simulink model "ros_image_filters_0704"  (R2017a)
settings: Solver=FixedStepDiscrete  StartTime=0.0  StopTime=inf  FixedStep=0.01  RelTol=1e-3  EnableMultiTasking=on
model workspace (MAT data in the model file):
  SL_ROS_VariableLengthArrays_MaxSizes.CommonInfo.ArrayTruncateAction = 'EmitWarning'
  SL_ROS_VariableLengthArrays_MaxSizes.MsgTypeMap = containers.Map
  SL_ROS_VariableLengthArrays_MaxSizes.MsgTypeMap.serialization.keys = {'sensor_msgs/Image'}
  SL_ROS_VariableLengthArrays_MaxSizes.MsgTypeMap.serialization.values{1}(1).PropertyName = 'Data'
  SL_ROS_VariableLengthArrays_MaxSizes.MsgTypeMap.serialization.values{1}(1).DataType = 'uint8'
  SL_ROS_VariableLengthArrays_MaxSizes.MsgTypeMap.serialization.values{1}(1).MaxLength = 1555200
  SL_ROS_VariableLengthArrays_MaxSizes.MsgTypeMap.serialization.values{1}(2).PropertyName = 'Encoding'
  SL_ROS_VariableLengthArrays_MaxSizes.MsgTypeMap.serialization.values{1}(2).DataType = 'uint8'
  SL_ROS_VariableLengthArrays_MaxSizes.MsgTypeMap.serialization.values{1}(2).MaxLength = 4
  SL_ROS_VariableLengthArrays_MaxSizes.MsgTypeMap.serialization.uniformity = 0
  SL_ROS_VariableLengthArrays_MaxSizes.MsgTypeMap.serialization.keyType = 'char'
  SL_ROS_VariableLengthArrays_MaxSizes.MsgTypeMap.serialization.valueType = 'any'
  blockSize = [270 480]
undefined symbols (not defined in the file): Rec, SDTV, strel
libraries: robotlib x7, visionconversions x5, visionsinks x5, simulink x3, visionmorphops x2, visionfilter x1, visionanalysis x1
settings Model: Creator=qifan  LastModifiedBy=qifan
settings SolverCC: AutoInsertRateTranBlk=on
settings DataIOCC: SaveOutput=off  SaveTime=off
settings OptimizationCC: PassReuseOutputArgsAs=Individual arguments  StateBitsets=on  DataBitsets=on  ZeroExternalMemoryAtStartup=off  ZeroInternalMemoryAtStartup=off  NoFixptDivByZeroProtection=on  LifeSpan=1  MaxStackSize=64
settings DebuggingCC: ParameterTunabilityLossMsg=error
settings HardwareCC: ProdBitPerPointer=32  ProdBitPerSizeT=32  ProdBitPerPtrDiffT=32  ProdLargestAtomicFloat=None  ProdIntDivRoundTo=Undefined  ProdEndianess=Unspecified  ProdWordSize=32  ProdHWDeviceType=Generic->Unspecified (assume 32-bit Generic)
settings SFSimCC: MATLABDynamicMemAlloc=off
settings RTWCC: SystemTargetFile=ert.tlc  HardwareBoard=Robot Operating System (ROS)  TLCOptions="-p0 -aInlineSetEventsForThisBaseRateFcn=TLC_FALSE -aSuppressMultiTaskScheduler=TLC_FALSE  -aRateBasedStepFcn=0"  GenCodeOnly=on  TemplateMakefile=ert_default_tmf  Description=Embedded Coder  GenerateReport=on  RTWVerbose=off  Toolchain=Catkin  IncludeHyperlinkInReport=on  LaunchReport=on  TargetLang=C++  GenerateTraceInfo=on  GenerateTraceReport=on  GenerateTraceReportSl=on  GenerateTraceReportSf=on  GenerateTraceReportEml=on
settings CodeAppCC: ForceParamTrailComments=on  IgnoreCustomStorageClasses=off  OperatorAnnotations=on  SimulinkDataObjDesc=on  SFDataObjDesc=on  MATLABFcnDesc=on  CustomSymbolStrGlobalVar=rt$N$M  CustomSymbolStrType=$N$M  CustomSymbolStrFcn=$N$M$F  CustomSymbolStrMacro=$N$M  InsertBlockDesc=on  MATLABSourceComments=on
settings ERTTargetCC: CodeReplacementLibrary=ISO_C  SupportNonFinite=off  SupportComplex=off  SupportContinuousTime=on  RootIOFormat=Structure reference

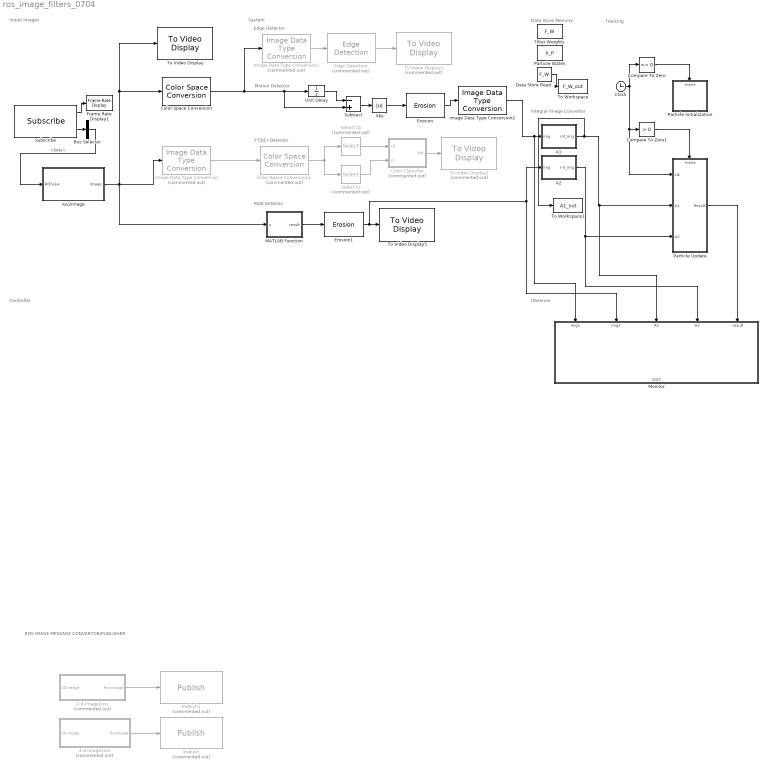
== system ros_image_filters_0704 ==
  note: Integral Image
      | Converter
  note: Observer
  note: Controller
  note: Imput Images
  note: System
  note: Y'CbCr Detector
  note: RGB Detector
  note: Edge Detector
  note: Motion Detector
  note: Data Store Memory
  note: Tracking
  note: ROS IMAGE MESSAGE CONVERTOR/PUBLISHER
  2-d-image2ros : Subsystem  Commented=on
  3-d-image2ros : Subsystem  Commented=on
  A1 : MATLAB Function  TreatAsAtomicUnit=on
  A2 : MATLAB Function  TreatAsAtomicUnit=on
  Abs : Abs
  Bus Selector : BusSelector  OutputSignals=Data
  Clock : Clock
  Color Classifier : Subsystem  Commented=on
  Color Space Conversion : visionconversions/Color Space  Conversion  conversion=Obsolete  conversionActive=R'G'B' to intensity  wp_str=D65  rec=Rec. 601 (SDTV)  sys=1125/60/2:1  imagePorts=One multidimensional signal
      settings: SourceProductName=Computer Vision System Toolbox
  Color Space Conversion1 : visionconversions/Color Space  Conversion  Commented=on  conversion=Obsolete  conversionActive=R'G'B' to Y'CbCr  wp_str=D65  rec=Rec. 601 (SDTV)  sys=1125/60/2:1  imagePorts=One multidimensional signal
      settings: SourceProductName=Computer Vision System Toolbox
  Compare To Zero : simulink/Logic and Bit Operations/Compare To Zero  relop=<=  OutDataTypeStr=boolean
  Compare To Zero1 : simulink/Logic and Bit Operations/Compare To Zero  relop=>  OutDataTypeStr=uint8
  Data Store Read : DataStoreRead  DataStoreName=F_W
  Edge Detection : visionanalysis/Edge Detection  Commented=on  method=Sobel  outputType=Binary image  userDefinedThreshold=off  thresholdSource=Input port  threshold=20  thresholdTuning=4  edgeThinning=off  threshold_canny=[0.25 0.60]  autoPercent=70  sigma=1  prodOutputMode=Binary point scaling  prodOutputWordLength=32  prodOutputFracLength=8  roundingMode=Floor  overflowMode=off
      settings: SourceProductName=Computer Vision System Toolbox  SourceProductBaseCode=VP
  Erosion : visionmorphops/Erosion  nhoodsrc=Specify via dialog  strel=strel('square',7)
      settings: SourceProductName=Computer Vision System Toolbox  SourceProductBaseCode=VP
  Erosion1 : visionmorphops/Erosion  nhoodsrc=Specify via dialog  strel=strel('square',7)
      settings: SourceProductName=Computer Vision System Toolbox  SourceProductBaseCode=VP
  Filter Weights : DataStoreMemory  DataStoreName=F_W  ReadBeforeWriteMsg=warning  WriteAfterWriteMsg=warning  WriteAfterReadMsg=warning  InitialValue=[0.5,0.5,0,0,0,0,0,0]  ShowAdditionalParam=off  OutDataTypeStr=double
  Frame Rate Display1 : visionsinks/Frame Rate Display  UpdateRate=10
      settings: SourceProductName=Computer Vision System Toolbox  SourceProductBaseCode=VP
  Image Data Type Conversion : visionconversions/Image Data Type Conversion  Commented=on  outDT=single  isSigned=on  wordLen=16  numFracBits=0
      settings: SourceProductName=Computer Vision System Toolbox  SourceProductBaseCode=VP
  Image Data Type Conversion1 : visionconversions/Image Data Type Conversion  Commented=on  outDT=single  isSigned=on  wordLen=16  numFracBits=0
      settings: SourceProductName=Computer Vision System Toolbox  SourceProductBaseCode=VP
  Image Data Type Conversion2 : visionconversions/Image Data Type Conversion  outDT=double  isSigned=on  wordLen=16  numFracBits=0
      settings: SourceProductName=Computer Vision System Toolbox  SourceProductBaseCode=VP
  MATLAB Function : MATLAB Function  TreatAsAtomicUnit=on
  Monitor : Subsystem
  Particle Initialization : Subsystem
  Particle States : DataStoreMemory  DataStoreName=X_P  ReadBeforeWriteMsg=warning  WriteAfterWriteMsg=warning  WriteAfterReadMsg=warning  InitialValue=zeros(200,3,2)  ShowAdditionalParam=off  OutDataTypeStr=double
  Particle Update : Subsystem
  Publish : robotlib/Publish  Commented=on  SourceLibraryInfo=This block requires Robotics System Toolbox  topicSource=Specify your own  topic=/image_color  messageType=sensor_msgs/Image  messageQueueLength=1
      settings: SourceProductBaseCode=RO
  Publish1 : robotlib/Publish  Commented=on  SourceLibraryInfo=This block requires Robotics System Toolbox  topicSource=Specify your own  topic=/image_erode  messageType=sensor_msgs/Image  messageQueueLength=1
      settings: SourceProductBaseCode=RO
  Select Cb : Selector  Commented=on  NumberOfDimensions=3  InputPortWidth=3  IndexOptions=Select all,Select all,Index vector (dialog)  Indices=[1 3],1,2  OutputSizes=1,1,1
  Select Cr : Selector  Commented=on  NumberOfDimensions=3  InputPortWidth=3  IndexOptions=Select all,Select all,Index vector (dialog)  Indices=[1 3],1,3  OutputSizes=1,1,1
  Subscribe : robotlib/Subscribe  SourceLibraryInfo=This block requires Robotics System Toolbox  topicSource=Specify your own  topic=/image_bridge  messageType=sensor_msgs/Image  sampleTime=-1  messageQueueLength=1
      settings: SourceProductBaseCode=RO
  Subtract : Sum  Inputs=-+
  To Video Display : visionsinks/To Video Display  windowSizeMode=Normal  openAtMdlStart=on  fullScreen=off  videoWindowX=160  videoWindowY=130  saveWindowSize=off  videoWindowWidth=960  videoWindowHeight=540  inputColorFormat=RGB  inputType=Obsolete  imagePorts=One multidimensional signal  OutputDevice=On-screen video monitor  dataOrg=Column-major  isWindowOpen=off
      settings: SourceProductName=Computer Vision System Toolbox
  To Video Display1 : visionsinks/To Video Display  Commented=on  windowSizeMode=Normal  openAtMdlStart=on  fullScreen=off  videoWindowX=260  videoWindowY=97  saveWindowSize=off  videoWindowWidth=962  videoWindowHeight=542  inputColorFormat=RGB  inputType=Obsolete  imagePorts=One multidimensional signal  OutputDevice=On-screen video monitor  dataOrg=Column-major  isWindowOpen=off
      settings: SourceProductName=Computer Vision System Toolbox
  To Video Display2 : visionsinks/To Video Display  Commented=on  windowSizeMode=Normal  openAtMdlStart=on  fullScreen=off  videoWindowX=184  videoWindowY=153  saveWindowSize=off  videoWindowWidth=960  videoWindowHeight=540  inputColorFormat=RGB  inputType=Obsolete  imagePorts=One multidimensional signal  OutputDevice=On-screen video monitor  dataOrg=Column-major  isWindowOpen=off
      settings: SourceProductName=Computer Vision System Toolbox
  To Video Display5 : visionsinks/To Video Display  windowSizeMode=Normal  openAtMdlStart=on  fullScreen=off  videoWindowX=260  videoWindowY=97  saveWindowSize=off  videoWindowWidth=962  videoWindowHeight=542  inputColorFormat=RGB  inputType=Obsolete  imagePorts=One multidimensional signal  OutputDevice=On-screen video monitor  dataOrg=Column-major  isWindowOpen=off
      settings: SourceProductName=Computer Vision System Toolbox
  To Workspace : ToWorkspace  VariableName=F_W_out  SaveFormat=Timeseries  SampleTime=-1
  To Workspace1 : ToWorkspace  VariableName=A1_out  SaveFormat=Timeseries  SampleTime=-1
  Unit Delay : UnitDelay  SampleTime=-1
  ros2image : Subsystem
  wires:
  Subscribe/1 -> Frame Rate Display1/1
  Bus Selector/1 -> ros2image/1(ROSraw)  "<Data>"
  Subscribe/2 -> Bus Selector/1
  Color Space Conversion/1 -> Unit Delay/1, Subtract/2, Image Data Type Conversion1/1
  3-d-image2ros/1(RosImage) -> Publish/1
  2-d-image2ros/1(Ros-image) -> Publish1/1
  Color Space Conversion1/1 -> Select Cr/1, Select Cb/1
  Select Cb/1 -> Color Classifier/1(cb)
  Select Cr/1 -> Color Classifier/2(cr)
  Color Classifier/1(BW) -> To Video Display1/1
  Image Data Type Conversion/1 -> Color Space Conversion1/1
  Edge Detection/1 -> To Video Display2/1
  Image Data Type Conversion1/1 -> Edge Detection/1
  Unit Delay/1 -> Subtract/1
  Subtract/1 -> Abs/1
  Abs/1 -> Erosion/1
  Erosion/1 -> Image Data Type Conversion2/1
  MATLAB Function/1(result) -> Erosion1/1
  Clock/1 -> Compare To Zero1/1, Particle Update/1(clk), Compare To Zero/1
  Compare To Zero/1 -> Particle Initialization/Enable
  Compare To Zero1/1 -> Particle Update/Enable
  Erosion1/1 -> A2/1(img), Monitor/2(img2), To Video Display5/1
  ros2image/1(Image) -> MATLAB Function/1(u), Image Data Type Conversion/1, Color Space Conversion/1, To Video Display/1
  Particle Update/1(Result) -> Monitor/5(result)
  A1/1(int_img) -> To Workspace1/1, Particle Update/2(A1), Monitor/3("A1 ")
  A2/1(int_img) -> Particle Update/3(A2), Monitor/4(A2)
  Image Data Type Conversion2/1 -> Monitor/1(img1), A1/1(img)
  Data Store Read/1 -> To Workspace/1

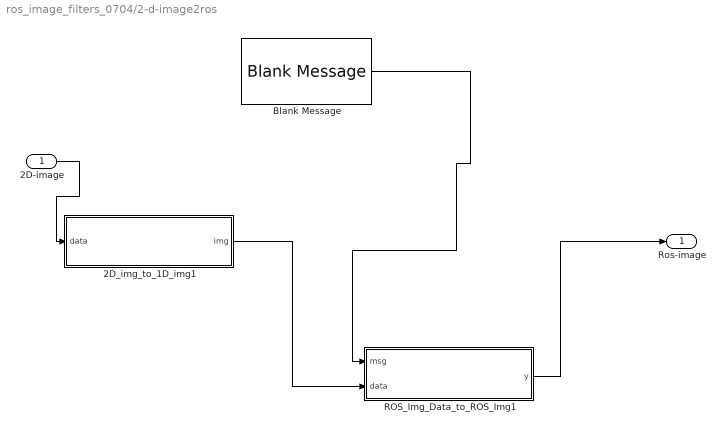
== system ros_image_filters_0704/2-d-image2ros ==
  2D-image : Inport
  2D_img_to_1D_img1 : MATLAB Function  TreatAsAtomicUnit=on
  Blank Message : robotlib/Blank Message  SourceLibraryInfo=This block requires Robotics System Toolbox  messageType=sensor_msgs/Image  SampleTime=inf
      settings: SourceProductBaseCode=RO
  ROS_Img_Data_to_ROS_Img1 : MATLAB Function  TreatAsAtomicUnit=on
  Ros-image : Outport
  wires:
  2D-image/1 -> 2D_img_to_1D_img1/1(data)
  ROS_Img_Data_to_ROS_Img1/1(y) -> Ros-image/1
  Blank Message/1 -> ROS_Img_Data_to_ROS_Img1/1(msg)
  2D_img_to_1D_img1/1(img) -> ROS_Img_Data_to_ROS_Img1/2(data)

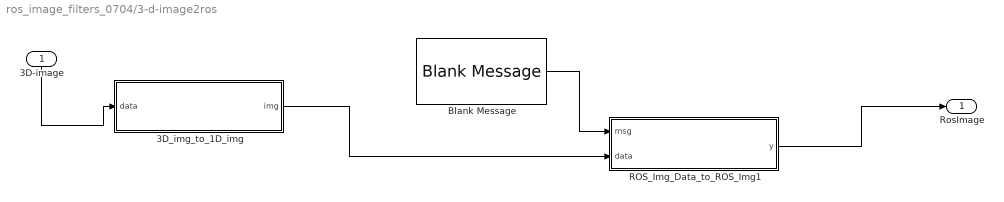
== system ros_image_filters_0704/3-d-image2ros ==
  3D-image : Inport
  3D_img_to_1D_img : MATLAB Function  TreatAsAtomicUnit=on
  Blank Message : robotlib/Blank Message  SourceLibraryInfo=This block requires Robotics System Toolbox  messageType=sensor_msgs/Image  SampleTime=inf
      settings: SourceProductBaseCode=RO
  ROS_Img_Data_to_ROS_Img1 : MATLAB Function  TreatAsAtomicUnit=on
  RosImage : Outport
  wires:
  3D-image/1 -> 3D_img_to_1D_img/1(data)
  ROS_Img_Data_to_ROS_Img1/1(y) -> RosImage/1
  Blank Message/1 -> ROS_Img_Data_to_ROS_Img1/1(msg)
  3D_img_to_1D_img/1(img) -> ROS_Img_Data_to_ROS_Img1/2(data)

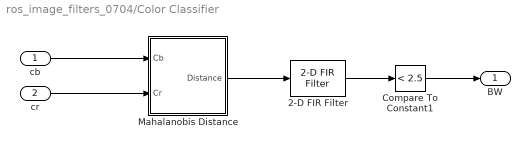
== system ros_image_filters_0704/Color Classifier ==
  cb : Inport
  cr : Inport  Port=2
  2-D FIR Filter : visionfilter/2-D FIR Filter  separable=off  filtSrc=Specify via dialog  filterMtrx=single(1/9*ones(3))  verticalFilter=[4 0]  horizontalFilter=[4 0]  outSize=Full  padType=Constant  padSrc=Specify via dialog  padVal=0  method=Convolution  firstCoeffSignedness=Signed  firstCoeffDataTypeStr=Inherit: Same word length as input  firstCoeffLastDataTypeStr=Inherit: Same word length as input  firstCoeffMin=[]  firstCoeffMax=[]  outputMode=Binary point scaling  outputWordLength=32  outputFracLength=12  outputSignedness=Auto  outputDataTypeStr=fixdt([],32,12)  outputLastDataTypeStr=fixdt([],32,12)  outputMin=[]  outputMax=[]  accumDataTypeStr=Inherit: Same as product output  accumLastDataTypeStr=Inherit: Same as product output  prodOutputMode=Binary point scaling  prodOutputWordLength=32  prodOutputFracLength=10  prodOutputDataTypeStr=fixdt([],32,10)  prodOutputLastDataTypeStr=fixdt([],32,10)  roundingMode=Floor  overflowMode=off
      settings: SourceProductName=Computer Vision System Toolbox  SourceProductBaseCode=VP
  Compare To Constant1 : simulink/Logic and Bit Operations/Compare To Constant  relop=<  const=2.5  OutDataTypeStr=boolean  ZeroCross=off
  "Mahalanobis Distance " : Subsystem
  BW : Outport
  wires:
  "Mahalanobis Distance "/1(Distance) -> 2-D FIR Filter/1
  cb/1 -> "Mahalanobis Distance "/1(Cb)
  cr/1 -> "Mahalanobis Distance "/2(Cr)
  Compare To Constant1/1 -> BW/1
  2-D FIR Filter/1 -> Compare To Constant1/1

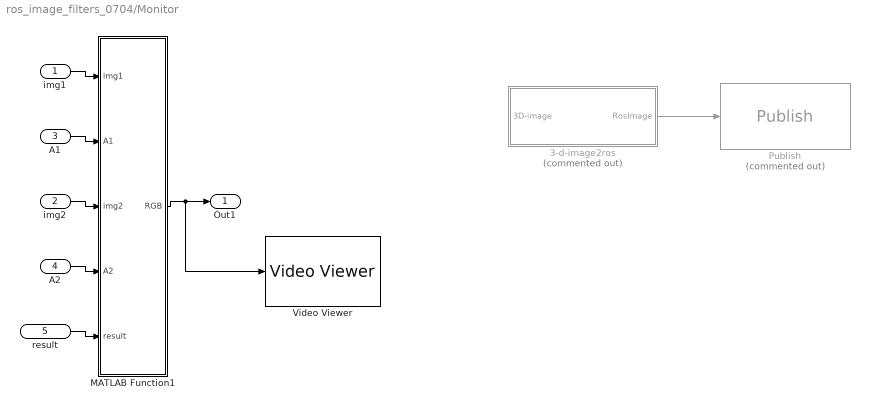
== system ros_image_filters_0704/Monitor ==
  img1 : Inport
  img2 : Inport  Port=2
  "A1 " : Inport  Port=3
  A2 : Inport  Port=4
  result : Inport  Port=5
  3-d-image2ros : Subsystem  Commented=on
  MATLAB Function1 : MATLAB Function  TreatAsAtomicUnit=on
  Publish : robotlib/Publish  Commented=on  SourceLibraryInfo=This block requires Robotics System Toolbox  topicSource=Specify your own  topic=/tracking_result  messageType=sensor_msgs/Image  messageQueueLength=1
      settings: SourceProductBaseCode=RO
  Video Viewer : VideoViewer  FigPos=[58 798 1223 693]
  Out1 : Outport
  wires:
  MATLAB Function1/1(RGB) -> Video Viewer/1, Out1/1
  result/1 -> MATLAB Function1/5(result)
  "A1 "/1 -> MATLAB Function1/2(A1)
  A2/1 -> MATLAB Function1/4(A2)
  img1/1 -> MATLAB Function1/1(img1)
  img2/1 -> MATLAB Function1/3(img2)
  3-d-image2ros/1(RosImage) -> Publish/1

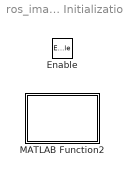
== system ros_image_filters_0704/Particle Initialization ==
  Enable : EnablePort
  MATLAB Function2 : MATLAB Function  TreatAsAtomicUnit=on

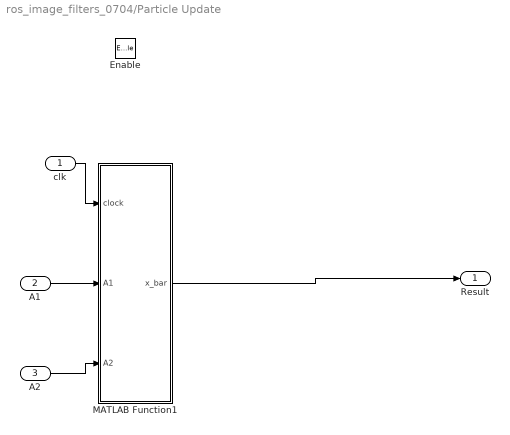
== system ros_image_filters_0704/Particle Update ==
  clk : Inport
  A1 : Inport  Port=2
  A2 : Inport  Port=3
  Enable : EnablePort
  MATLAB Function1 : MATLAB Function  TreatAsAtomicUnit=on
  Result : Outport
  wires:
  clk/1 -> MATLAB Function1/1(clock)
  MATLAB Function1/1(x_bar) -> Result/1
  A1/1 -> MATLAB Function1/2(A1)
  A2/1 -> MATLAB Function1/3(A2)

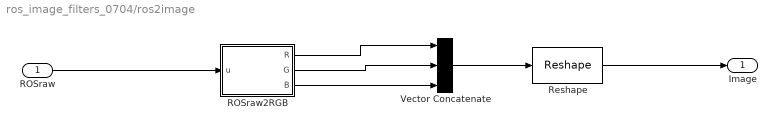
== system ros_image_filters_0704/ros2image ==
  ROSraw : Inport  PortDimensions=1555200
  ROSraw2RGB : MATLAB Function  TreatAsAtomicUnit=on
  Reshape : Reshape  OutputDimensionality=Customize  OutputDimensions=[540,960,3]
  Vector Concatenate : Concatenate  NumInputs=3  Mode=Multidimensional array  ConcatenateDimension=2
  Image : Outport
  wires:
  ROSraw2RGB/3(B) -> Vector Concatenate/3
  ROSraw2RGB/1(R) -> Vector Concatenate/1
  Reshape/1 -> Image/1
  ROSraw/1 -> ROSraw2RGB/1(u)
  ROSraw2RGB/2(G) -> Vector Concatenate/2
  Vector Concatenate/1 -> Reshape/1

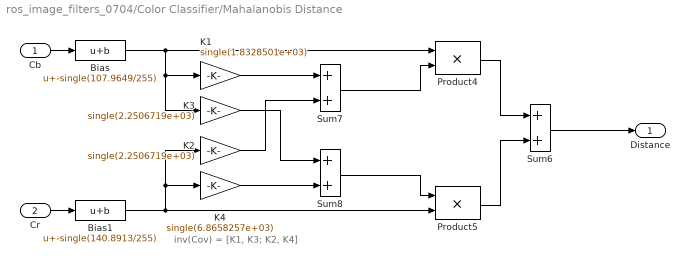
== system ros_image_filters_0704/Color Classifier/Mahalanobis Distance  ==
  note: inv(Cov) = [K1, K3; K2, K4]
  Cb : Inport
  Cr : Inport  Port=2
  Bias : Bias  Bias=-single(107.9649/255)
  Bias1 : Bias  Bias=-single(140.8913/255)
  K1 : Gain  Gain=single(1.8328501e+03)  SaturateOnIntegerOverflow=on  OutDataTypeStr=Inherit: Same as input  ParamDataTypeStr=Inherit: Same as input
  K2 : Gain  Gain=single(2.2506719e+03)  SaturateOnIntegerOverflow=on  OutDataTypeStr=Inherit: Same as input  ParamDataTypeStr=Inherit: Same as input
  K3 : Gain  Gain=single(2.2506719e+03)  SaturateOnIntegerOverflow=on  OutDataTypeStr=Inherit: Same as input  ParamDataTypeStr=Inherit: Same as input
  K4 : Gain  Gain=single(6.8658257e+03)  SaturateOnIntegerOverflow=on  OutDataTypeStr=Inherit: Same as input  ParamDataTypeStr=Inherit: Same as input
  Product4 : Product  SaturateOnIntegerOverflow=on  InputSameDT=on  OutDataTypeStr=Inherit: Same as first input
  Product5 : Product  SaturateOnIntegerOverflow=on  InputSameDT=on  OutDataTypeStr=Inherit: Same as first input
  Sum6 : Sum  SaturateOnIntegerOverflow=on  InputSameDT=on  OutDataTypeStr=Inherit: Same as first input
  Sum7 : Sum  SaturateOnIntegerOverflow=on  InputSameDT=on  OutDataTypeStr=Inherit: Same as first input
  Sum8 : Sum  SaturateOnIntegerOverflow=on  InputSameDT=on  OutDataTypeStr=Inherit: Same as first input
  Distance : Outport
  wires:
  Cb/1 -> Bias/1
  Cr/1 -> Bias1/1
  K4/1 -> Sum8/2
  Product4/1 -> Sum6/1
  Product5/1 -> Sum6/2
  K1/1 -> Sum7/1
  K2/1 -> Sum7/2
  K3/1 -> Sum8/1
  Sum7/1 -> Product4/2
  Sum8/1 -> Product5/1
  Bias/1 -> Product4/1, K1/1, K3/1
  Bias1/1 -> Product5/2, K4/1, K2/1
  Sum6/1 -> Distance/1

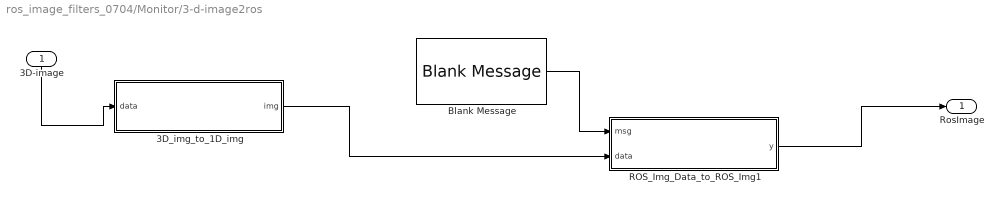
== system ros_image_filters_0704/Monitor/3-d-image2ros ==
  3D-image : Inport
  3D_img_to_1D_img : MATLAB Function  TreatAsAtomicUnit=on
  Blank Message : robotlib/Blank Message  SourceLibraryInfo=This block requires Robotics System Toolbox  messageType=sensor_msgs/Image  SampleTime=inf
      settings: SourceProductBaseCode=RO
  ROS_Img_Data_to_ROS_Img1 : MATLAB Function  TreatAsAtomicUnit=on
  RosImage : Outport
  wires:
  3D-image/1 -> 3D_img_to_1D_img/1(data)
  ROS_Img_Data_to_ROS_Img1/1(y) -> RosImage/1
  Blank Message/1 -> ROS_Img_Data_to_ROS_Img1/1(msg)
  3D_img_to_1D_img/1(img) -> ROS_Img_Data_to_ROS_Img1/2(data)

== matlab function ros_image_filters_0704/3-d-image2ros/ROS_Img_Data_to_ROS_Img1 ==
  data: msg input; y output Bus: SL_Bus_ros_image_filters_0619_sensor_msgs_Image; data input size=1555200
function y = rosImgData2rosImg(msg, data)
% assignString - Assign a string in a ROS message
%
% MSG = assignString(blankMsg) assigns a known string value to a 
%  string field in a ROS message, and outputs the updated ROS message.
%
%  blankMsg (input): A bus for a 'std_msgs/String' message. This is 
%      used to initialize the output. 
%  msg (output): A bus for a 'std_msgs/String' message, with the Data 
%      field set to a string.

%   Copyright 2015 The MathWorks, Inc.
%#codegen

% Note: The datatype of 'msg' has been explicitly set to the appropriate 
% Simulink bus type ("Bus: SL_Bus_robotROSMessageUsageExample_std_msgs_String"). 
%
% If the model name is changed, the datatype needs to be changed as well:
%   1) Click "Edit Data" in the Editor toolstrip to open "Ports and Data Manager"
%   2) Select "msg". From the "Type" dropdown, select "--- Refresh data types ---"
%   3) Set datatype to "Bus: SL_Bus_<modelname>_std_msgs_String"
    
stringToAssign = 'rgb8';
height = 540;
width = 960;

% msg (std_msgs/String) consists of
%           Data : array of type uint8
%   Data_SL_Info : struct with fields CurrentLength, ReceivedLength
msg.Encoding = uint8(stringToAssign)';
msg.Encoding_SL_Info.CurrentLength = uint32(length(stringToAssign));

msg.Data = uint8(data);
msg.Data_SL_Info.CurrentLength = uint32(length(data));

msg.Height = uint32(height);
msg.Width = uint32(width);
msg.Step = uint32(width * 3);

y = msg;

== matlab function ros_image_filters_0704/3-d-image2ros/3D_img_to_1D_img ==
  data: img output uint8; data input
function img = threeD_img_to_1D_img(data)
% assignString - Assign a string in a ROS message
%
% MSG = assignString(blankMsg) assigns a known string value to a 
%  string field in a ROS message, and outputs the updated ROS message.
%
%  blankMsg (input): A bus for a 'std_msgs/String' message. This is 
%      used to initialize the output. 
%  msg (output): A bus for a 'std_msgs/String' message, with the Data 
%      field set to a string.

%   Copyright 2015 The MathWorks, Inc.
%#codegen

% Note: The datatype of 'msg' has been explicitly set to the appropriate 
% Simulink bus type ("Bus: SL_Bus_robotROSMessageUsageExample_std_msgs_String"). 
%
% If the model name is changed, the datatype needs to be changed as well:
%   1) Click "Edit Data" in the Editor toolstrip to open "Ports and Data Manager"
%   2) Select "msg". From the "Type" dropdown, select "--- Refresh data types ---"
%   3) Set datatype to "Bus: SL_Bus_<modelname>_std_msgs_String"
    

% msg (std_msgs/String) consists of
%           Data : array of type uint8
%   Data_SL_Info : struct with fields CurrentLength, ReceivedLength
img = uint8(zeros(1, 1555200));
img(1:3:end) = data(:,:,1)';
img(2:3:end) = data(:,:,2)';
img(3:3:end) = data(:,:,3)';

== matlab function ros_image_filters_0704/MATLAB Function ==
  data: u input; result output
function result = fcn(u)

R = u(:, :, 1);
G = u(:, :, 2);
B = u(:, :, 3);


result = double(zeros(540, 960, 1));

%result(:, :, 1) = R./(R + G + B);
%result(:, :, 2) = G./(R + G + B);
%result(:, :, 3) = B./(R + G + B);


for i = 1:540
    for j = 1:960
        rgb = u(i, j, :);
        if rgb(1) > 95 && rgb(2) > 40 && rgb(3) > 20 && max(rgb) - min(rgb) > 15 ...
            && abs(rgb(1) - rgb(2)) > 15 && rgb(1) > rgb(2) && rgb(1) > rgb(3)
            result(i, j) = 1;
        end
    end
end

== matlab function ros_image_filters_0704/2-d-image2ros/2D_img_to_1D_img1 ==
  data: img output uint8; data input
function img = twoD_img_to_1D_img(data)
% assignString - Assign a string in a ROS message
%
% MSG = assignString(blankMsg) assigns a known string value to a 
%  string field in a ROS message, and outputs the updated ROS message.
%
%  blankMsg (input): A bus for a 'std_msgs/String' message. This is 
%      used to initialize the output. 
%  msg (output): A bus for a 'std_msgs/String' message, with the Data 
%      field set to a string.

%   Copyright 2015 The MathWorks, Inc.
%#codegen

% Note: The datatype of 'msg' has been explicitly set to the appropriate 
% Simulink bus type ("Bus: SL_Bus_robotROSMessageUsageExample_std_msgs_String"). 
%
% If the model name is changed, the datatype needs to be changed as well:
%   1) Click "Edit Data" in the Editor toolstrip to open "Ports and Data Manager"
%   2) Select "msg". From the "Type" dropdown, select "--- Refresh data types ---"
%   3) Set datatype to "Bus: SL_Bus_<modelname>_std_msgs_String"
    

% msg (std_msgs/String) consists of
%           Data : array of type uint8
%   Data_SL_Info : struct with fields CurrentLength, ReceivedLength
img = uint8(zeros(1, 1555200));
img(1:3:end) = data';
img(2:3:end) = data';
img(3:3:end) = data';

== matlab function ros_image_filters_0704/2-d-image2ros/ROS_Img_Data_to_ROS_Img1 ==
  data: msg input; y output Bus: SL_Bus_ros_image_filters_0619_sensor_msgs_Image; data input size=1555200
function y = rosImgData2rosImg(msg, data)
% assignString - Assign a string in a ROS message
%
% MSG = assignString(blankMsg) assigns a known string value to a 
%  string field in a ROS message, and outputs the updated ROS message.
%
%  blankMsg (input): A bus for a 'std_msgs/String' message. This is 
%      used to initialize the output. 
%  msg (output): A bus for a 'std_msgs/String' message, with the Data 
%      field set to a string.

%   Copyright 2015 The MathWorks, Inc.
%#codegen

% Note: The datatype of 'msg' has been explicitly set to the appropriate 
% Simulink bus type ("Bus: SL_Bus_robotROSMessageUsageExample_std_msgs_String"). 
%
% If the model name is changed, the datatype needs to be changed as well:
%   1) Click "Edit Data" in the Editor toolstrip to open "Ports and Data Manager"
%   2) Select "msg". From the "Type" dropdown, select "--- Refresh data types ---"
%   3) Set datatype to "Bus: SL_Bus_<modelname>_std_msgs_String"
    
stringToAssign = 'rgb8';
height = 540;
width = 960;

% msg (std_msgs/String) consists of
%           Data : array of type uint8
%   Data_SL_Info : struct with fields CurrentLength, ReceivedLength
msg.Encoding = uint8(stringToAssign)';
msg.Encoding_SL_Info.CurrentLength = uint32(length(stringToAssign));

msg.Data = uint8(data);
msg.Data_SL_Info.CurrentLength = uint32(length(data));

msg.Height = uint32(height);
msg.Width = uint32(width);
msg.Step = uint32(width * 3);

y = msg;

== matlab function ros_image_filters_0704/ros2image/ROSraw2RGB ==
  data: u input; R output; G output; B output
function [R,G,B] = fcn(u)
%#codegen
Rs = u(1:3:end);
Gs = u(2:3:end);
Bs = u(3:3:end);
B = reshape(Rs,960,540)';
G = reshape(Gs,960,540)';
R = reshape(Bs,960,540)';

== matlab function ros_image_filters_0704/Particle Update/MATLAB Function1 ==
  data: clock input; X_P data_store_memory; x_bar output; A1 input; A2 input
function x_bar = fcn(clock,A1,A2)

coder.extrinsic('imshow');
global X_P;


N = 200; % sample population

W_pre = X_P(:, 3, 2); % weights of old sample
S_new = zeros(N, 3, 2); % initial new sample container

s_k_pre = randsample(N,N,true,W_pre); % Sampling from previous state

%disp(s_k_pre);

for i = 1:N
    index = s_k_pre(i);
    p_top_left = reshape(X_P(index, 1, :), [1 2]); % get sample position
    
    s_v = reshape(X_P(index, 2, :),[1 2]);% get sample velocity
    s_width = X_P(index, 3, 1);% get sample width
    
    p_inrange_1 = [1, 1] < p_top_left;
    p_inrange_2 = p_top_left <= [540 - s_width, 960 - s_width];
    if sum([p_inrange_1 p_inrange_2]) ~= 4
        p_top_left = [rand * (540 - s_width), rand * (960 - s_width)];
    end

    p_tl = ceil(p_top_left);
    p_tr = ceil(p_top_left + [0, s_width]);
    p_bl = ceil(p_top_left + [s_width, 0]);
    p_br = ceil(p_top_left + [s_width, s_width]);
    
    value = A1(p_tl(1), p_tl(2)) + A1(p_br(1),p_br(2))...
    - A1(p_tr(1), p_tr(2)) - A1(p_bl(1),p_bl(2)); % update new weight

    w_new = value;
    
    if value < 1
        p_top_left = [rand * (540 - s_width), rand * (960 - s_width)];
        w_new = value + 0.01;
    end
    
    s_v_new = s_v + [randn, randn] * 5; % update velocity
    % s_width_new = s_width + randn; % update width
    p_new = p_top_left + s_v + randn;
    
    S_new(i, :, :) = [p_new; s_v_new; s_width, w_new];
end



[~, max_index] = max(X_P(:, 3, 2));
%RGB = insertMarker(image,int16(reshape([S_new(:,1,2), S_new(:,1,1)], [200, 2])),'o','color',[255 0 0],...
%    'size', 10);
%%% !!!!!!!!!!!!!!RGB = insertShape(img1, 'FilledCircle', [int16([S_new(max_index, 1, 2), S_new(max_index, 1, 1)]),10]);
x_bar = reshape(X_P(max_index, :, :), [3 2]);
X_P = S_new;
%disp(x_bar);
%disp(size(x_bar));


%RGB = insertMarker(RGB, reshape([S_new(:,1,2),S_new(:,1,1)], [N 2]),'o','color','green','size',10);


%imshow(image);
%hold on;
%[max_weight max_index] = max(S_new(:, 3, 2));
%plot(S_new(:,1,2),S_new(:,1,1),'r.','MarkerSize',20);
%plot(S_new(max_index, 1, 2), S_new(max_index, 1, 1), 'g.', 'MarkerSize', 100);
%hold off;

== matlab function ros_image_filters_0704/Particle Initialization/MATLAB Function2 ==
  data: X_P data_store_memory
function fcn

global X_P;


N = 200;


for i = 1:N
    weight = 1 / N;
    width = 50;
    
    X_P(i,2,:) = [0, 0];
    X_P(i,3,:) = [width, weight];
    x = rand * 540;
    y = rand * 960;
    X_P(i,1,:) = [x, y];
end

== matlab function ros_image_filters_0704/Monitor/3-d-image2ros/3D_img_to_1D_img ==
  data: img output uint8; data input
function img = threeD_img_to_1D_img(data)
% assignString - Assign a string in a ROS message
%
% MSG = assignString(blankMsg) assigns a known string value to a 
%  string field in a ROS message, and outputs the updated ROS message.
%
%  blankMsg (input): A bus for a 'std_msgs/String' message. This is 
%      used to initialize the output. 
%  msg (output): A bus for a 'std_msgs/String' message, with the Data 
%      field set to a string.

%   Copyright 2015 The MathWorks, Inc.
%#codegen

% Note: The datatype of 'msg' has been explicitly set to the appropriate 
% Simulink bus type ("Bus: SL_Bus_robotROSMessageUsageExample_std_msgs_String"). 
%
% If the model name is changed, the datatype needs to be changed as well:
%   1) Click "Edit Data" in the Editor toolstrip to open "Ports and Data Manager"
%   2) Select "msg". From the "Type" dropdown, select "--- Refresh data types ---"
%   3) Set datatype to "Bus: SL_Bus_<modelname>_std_msgs_String"
    

% msg (std_msgs/String) consists of
%           Data : array of type uint8
%   Data_SL_Info : struct with fields CurrentLength, ReceivedLength
img = uint8(zeros(1, 1555200));
img(1:3:end) = data(:,:,1)';
img(2:3:end) = data(:,:,2)';
img(3:3:end) = data(:,:,3)';

== matlab function ros_image_filters_0704/Monitor/3-d-image2ros/ROS_Img_Data_to_ROS_Img1 ==
  data: msg input; y output Bus: SL_Bus_ros_image_filters_0703_sensor_msgs_Image; data input size=1555200
function y = rosImgData2rosImg(msg, data)
% assignString - Assign a string in a ROS message
%
% MSG = assignString(blankMsg) assigns a known string value to a 
%  string field in a ROS message, and outputs the updated ROS message.
%
%  blankMsg (input): A bus for a 'std_msgs/String' message. This is 
%      used to initialize the output. 
%  msg (output): A bus for a 'std_msgs/String' message, with the Data 
%      field set to a string.

%   Copyright 2015 The MathWorks, Inc.
%#codegen

% Note: The datatype of 'msg' has been explicitly set to the appropriate 
% Simulink bus type ("Bus: SL_Bus_robotROSMessageUsageExample_std_msgs_String"). 
%
% If the model name is changed, the datatype needs to be changed as well:
%   1) Click "Edit Data" in the Editor toolstrip to open "Ports and Data Manager"
%   2) Select "msg". From the "Type" dropdown, select "--- Refresh data types ---"
%   3) Set datatype to "Bus: SL_Bus_<modelname>_std_msgs_String"
    
stringToAssign = 'rgb8';
height = 540;
width = 960;

% msg (std_msgs/String) consists of
%           Data : array of type uint8
%   Data_SL_Info : struct with fields CurrentLength, ReceivedLength
msg.Encoding = uint8(stringToAssign)';
msg.Encoding_SL_Info.CurrentLength = uint32(length(stringToAssign));

msg.Data = uint8(data);
msg.Data_SL_Info.CurrentLength = uint32(length(data));

msg.Height = uint32(height);
msg.Width = uint32(width);
msg.Step = uint32(width * 3);

y = msg;

== matlab function ros_image_filters_0704/Monitor/MATLAB Function1 ==
  data: img1 input; A1 input; img2 input; A2 input; result input; RGB output size=[540 960 3]; F_W data_store_memory
function RGB = fcn(img1, A1, img2, A2, result)

global F_W;



% img_inputs = {img1, img2};
A_inputs = {A1, A2};


filter_size = 2;
filter_weights = zeros(filter_size, 1);

theta_min = 60;

x_position = result(1,:);
x_width = result(3,1);
x_weight = result(3,2);


if x_weight > theta_min
    weight_sum = 0;
    for i = 1:filter_size
        avg_val = mean(mean(A_inputs{i}));
        disp('avg_val:');
        disp(avg_val);
        disp('eval:');
        disp(eval_at_p(A_inputs{i}, x_position, x_width));
        filter_weights(i) = max(0.01, eval_at_p(A_inputs{i}, x_position, x_width)-avg_val);
    end
    disp('filter____weights:');
    disp(filter_weights);
    for i = 1:filter_size
        weight_sum = weight_sum + filter_weights(i);
    end
    for i = 1:filter_size
        F_W(i) = filter_weights(i)/weight_sum;
    end
    disp('filter weights:');
    disp([F_W(1), F_W(2)]);
else
    disp('filter weight reset');
    for i = 1:filter_size
        F_W(i) = 1/filter_size; 
    end
end

RGB = insertShape(img1, 'FilledCircle', [int16([result(1,2), result(1,1)]),10]);

end
%% the eval() function
function value = eval_at_p(A, point, width)
    p_tl = ceil([min(max(point(1),1), 541), min(max(point(2), 1), 961)]);
    p_tr = ceil([min(max(point(1),1), 541), max(min(point(2), 961 - width) + width, 1)]);
    p_bl = ceil([max(min(point(1),541 - width) + width, 1), min(max(point(2), 1), 961)]);
    p_br = ceil([max(min(point(1),541 - width) + width, 1), max(min(point(2),961 - width) + width, 1)]);
    
    value = A(p_tl(1), p_tl(2)) + A(p_br(1),p_br(2))...
    - A(p_tr(1), p_tr(2)) - A(p_bl(1),p_bl(2));
end

== matlab function ros_image_filters_0704/A1 ==
  data: img input; int_img output
function int_img = toIntImg(img)

int_img = integralImage(img);

== matlab function ros_image_filters_0704/A2 ==
  data: img input; int_img output
function int_img = toIntImg(img)

int_img = integralImage(img);
